simulink model "fourth"  (R2020a)
settings: Solver=VariableStepAuto  StartTime=0.0  StopTime=10.0  RelTol=1e-3
model workspace (MAT data in the model file):
  A = Simulink.Parameter
  A.Value = 0.25
  A.DataType = 'auto'
  A.Dimensions = [1 1]
  B = Simulink.Parameter
  B.Value = 0.5
  B.DataType = 'auto'
  B.Dimensions = [1 1]
  C = Simulink.Parameter
  C.Value = 0.4
  C.DataType = 'auto'
  C.Dimensions = [1 1]
  X = Simulink.Parameter
  X.Value = 1
  X.DataType = 'auto'
  X.Dimensions = [1 1]
settings Model: Creator=Admin  LastModifiedBy=Admin

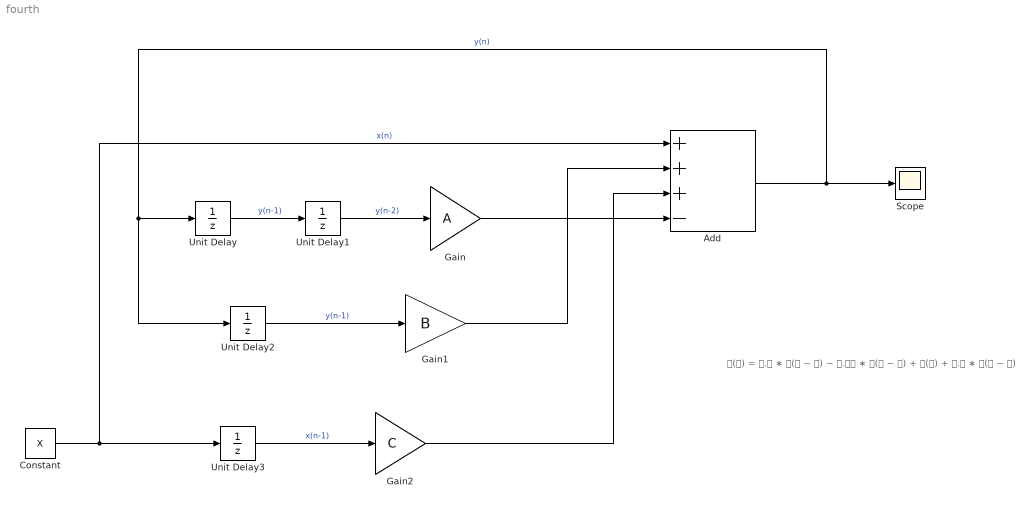
== system fourth ==
  note: 𝐲(𝐧) = 𝟎.𝟓 ∗ 𝐲(𝐧 − 𝟏) − 𝟎.𝟐𝟓 ∗ 𝐲(𝐧 − 𝟐) + 𝐱(𝐧) + 𝟎.𝟒 ∗ 𝐱(𝐧 − 𝟏)
  Add : Sum  Inputs=+++-
  Constant : Constant  Value=X
  Gain : Gain  Gain=A
  Gain1 : Gain  Gain=B
  Gain2 : Gain  Gain=C
  Scope : Scope
  Unit Delay{,1..3} (4 alike) : UnitDelay  SampleTime=-1  HasFrameUpgradeWarning=on
  wires:
  Unit Delay1/1 -> Gain/1  "y(n-2)"
  Unit Delay/1 -> Unit Delay1/1  "y(n-1)"
  Constant/1 -> Unit Delay3/1, Add/1  "x(n)"
  Add/1 -> Scope/1, Unit Delay/1, Unit Delay2/1  "y(n)"
  Gain/1 -> Add/4
  Unit Delay3/1 -> Gain2/1  "x(n-1)"
  Gain2/1 -> Add/3
  Unit Delay2/1 -> Gain1/1  "y(n-1)"
  Gain1/1 -> Add/2
